simulink model "heart"  (R2017b)
settings: Solver=VariableStepAuto  StartTime=0.0  StopTime=10  MaxStep=0.01  RelTol=1e-3
settings Model: Creator=prave  LastModifiedBy=prave

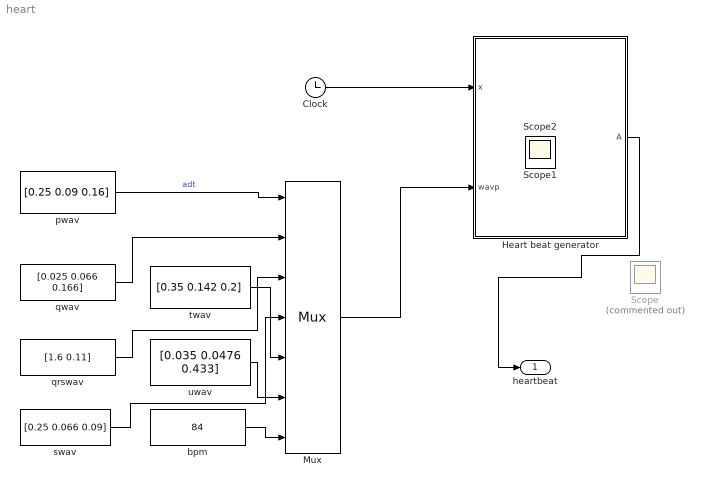
== system heart ==
  Clock : Clock
  Heart beat generator : MATLAB Function  TreatAsAtomicUnit=on
  Mux : Mux  Inputs=7
  Scope : Scope  Commented=on
  bpm : Constant  Value=84
  pwav : Constant  Value=[0.25 0.09 0.16]
  qrswav : Constant  Value=[1.6 0.11]
  qwav : Constant  Value=[0.025 0.066 0.166]
  swav : Constant  Value=[0.25 0.066 0.09]
  twav : Constant  Value=[0.35 0.142 0.2]
  uwav : Constant  Value=[0.035 0.0476 0.433]
  heartbeat : Outport
  Scope1 : Scope
  Scope2 : Scope
  wires:
  Clock/1 -> Heart beat generator/1(x)
  Heart beat generator/1(A) -> heartbeat/1
  pwav/1 -> Mux/1  "adt"
  bpm/1 -> Mux/7
  Mux/1 -> Heart beat generator/2(wavp)
  qwav/1 -> Mux/2
  qrswav/1 -> Mux/3
  swav/1 -> Mux/4
  twav/1 -> Mux/5
  uwav/1 -> Mux/6

== matlab function heart/Heart beat generator ==
  data: x input; A output; wavp input
function A = heartbeat(x,wavp)
     li=30/wavp(18);  
      
      a_pwav=wavp(1);
      d_pwav=wavp(2);
      t_pwav=wavp(3);  
     
      a_qwav=wavp(4);
      d_qwav=wavp(5);
      t_qwav=wavp(6);
      
      a_qrswav=wavp(7);
      d_qrswav=wavp(8);
      
      a_swav=wavp(9);
      d_swav=wavp(10);
      t_swav=wavp(11);
      
      a_twav=wavp(12);
      d_twav=wavp(13);
      t_twav=wavp(14);
      
      a_uwav=wavp(15);
      d_uwav=wavp(16);
      t_uwav=wavp(17);

       pwav=p_wav(x,a_pwav,d_pwav,t_pwav,li);

 
 %qwav output
 qwav=q_wav(x,a_qwav,d_qwav,t_qwav,li);

    
 %qrswav output
 qrswav=qrs_wav(x,a_qrswav,d_qrswav,li);

 %swav output
 swav=s_wav(x,a_swav,d_swav,t_swav,li);

 
 %twav output
 twav=t_wav(x,a_twav,d_twav,t_twav,li);

 
 %uwav output
 uwav=u_wav(x,a_uwav,d_uwav,t_uwav,li);

 %ecg output
 ecg=pwav+qrswav+twav+swav+qwav+uwav;
A = ecg ;
